simulink library "Tube_Alpha_sf"  (R2019b)
settings: Solver=ode45  StartTime=0.0  StopTime=10.0  RelTol=1e-3  EnableMultiTasking=on
undefined symbols (not defined in the file): Tube
libraries: simulink x1
settings Model: Creator=mbrauer  LastModifiedBy=bhisma
settings DataIOCC: LimitDataPoints=on  SaveFormat=Array  SignalLoggingSaveFormat=ModelDataLogs  ReturnWorkspaceOutputs=off
settings OptimizationCC: LifeSpan=inf
settings DebuggingCC: UnderspecifiedInitializationDetection=Classic  MergeDetectMultiDrivingBlocksExec=none  SolverPrmCheckMsg=warning  MultiTaskDSMMsg=warning  MultiTaskCondExecSysMsg=none  SFUnexpectedBacktrackingDiag=warning  SFNoUnconditionalDefaultTransitionDiag=warning  SFExecutionAtInitializationDiag=none  ArithmeticOperatorsInVariantConditions=warning
settings HardwareCC: ProdBitPerPointer=32  ProdBitPerSizeT=32  ProdBitPerPtrDiffT=32  ProdLargestAtomicFloat=None  ProdIntDivRoundTo=Undefined  ProdEndianess=Unspecified  ProdWordSize=32  ProdHWDeviceType=32-bit Generic
settings ModelReferenceCC: PropagateSignalLabelsOutOfModel=off
settings SFSimCC: SimUseLocalCustomCode=off  CustomCodeUndefinedFunction=UseInterfaceOnly
settings RTWCC: RTWUseLocalCustomCode=off
settings CodeAppCC: StateflowObjectComments=on
settings GRTTargetCC: TargetLangStandard=C89/C90 (ANSI)  GeneratePreprocessorConditionals=Disable all
settings ConfigComp: CovMetricSettings=dw  CovHtmlReporting=on  CovSaveCumulativeToWorkspaceVar=on  CovSaveSingleToWorkspaceVar=on  CovExternalEMLEnable=off

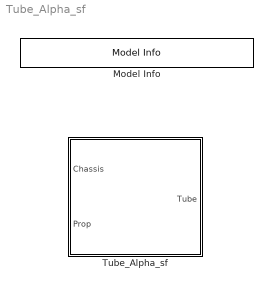
== system Tube_Alpha_sf ==
  Model Info : simulink/Model-Wide Utilities/Model Info  Frame=on  DisplayStringWithTags=Copyright 2013-2014 The MathWorks, Inc.  HorizontalTextAlignment=Center  LeftAlignmentValue=0.5
  Tube_Alpha_sf : Subsystem  VariantControl=VAR_Tube_Alpha

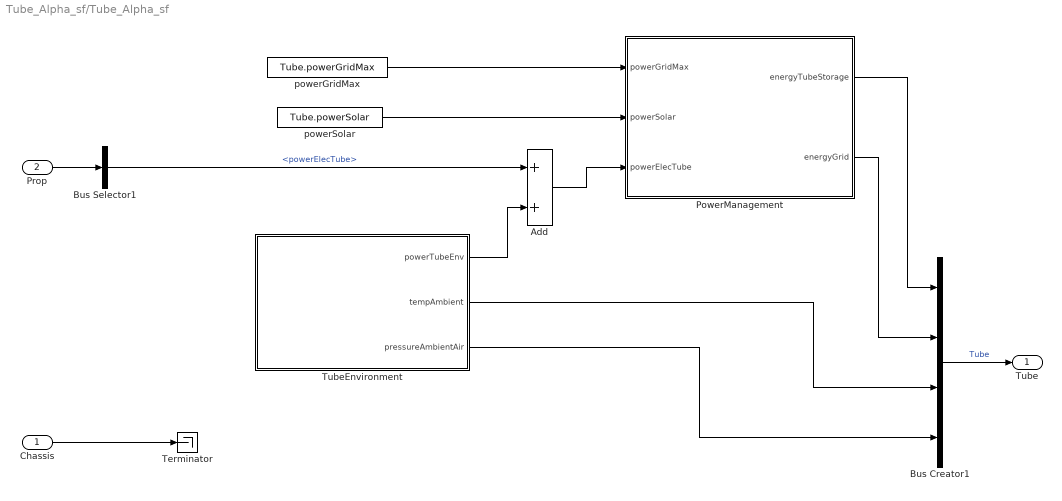
== system Tube_Alpha_sf/Tube_Alpha_sf ==
  Chassis : Inport
  Prop : Inport  Port=2
  Add : Sum
  Bus Creator1 : BusCreator  Inputs=4  NonVirtualBus=on
  Bus Selector1 : BusSelector  OutputSignals=powerElecTube
  PowerManagement : Subsystem
  Terminator : Terminator
  TubeEnvironment : Subsystem
  powerGridMax : Constant  Value=Tube.powerGridMax
  powerSolar : Constant  Value=Tube.powerSolar
  Tube : Outport
  wires:
  TubeEnvironment/2(tempAmbient) -> Bus Creator1/3
  Bus Creator1/1 -> Tube/1  "Tube"
  PowerManagement/1(energyTubeStorage) -> Bus Creator1/1
  Prop/1 -> Bus Selector1/1
  TubeEnvironment/1(powerTubeEnv) -> Add/2
  PowerManagement/2(energyGrid) -> Bus Creator1/2
  TubeEnvironment/3(pressureAmbientAir) -> Bus Creator1/4
  powerSolar/1 -> PowerManagement/2(powerSolar)
  powerGridMax/1 -> PowerManagement/1(powerGridMax)
  Bus Selector1/1 -> Add/1  "<powerElecTube>"
  Add/1 -> PowerManagement/3(powerElecTube)
  Chassis/1 -> Terminator/1

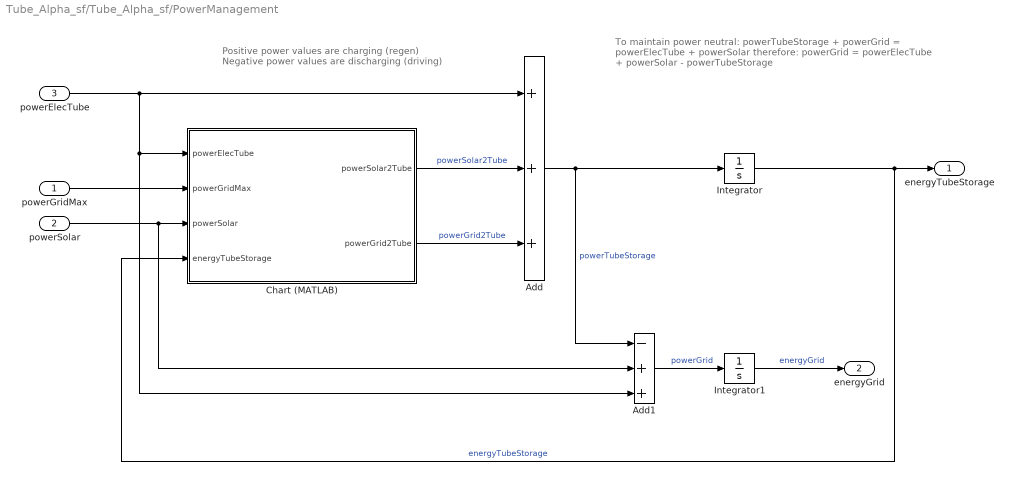
== system Tube_Alpha_sf/Tube_Alpha_sf/PowerManagement ==
  note: To maintain power neutral:
      | powerTubeStorage + powerGrid = powerElecTube + powerSolar
      |
      | therefore:
      | powerGrid = powerElecTube + powerSolar - powerTubeStorage
  note: Positive power values are charging (regen)
      | Negative power values are discharging (driving)
  powerGridMax : Inport
  powerSolar : Inport  Port=2
  powerElecTube : Inport  Port=3
  Add : Sum  Inputs=+++
  Add1 : Sum  Inputs=-++
  Chart (MATLAB) : Stateflow chart  TreatAsAtomicUnit=on
  Integrator : Integrator  InitialCondition=Tube.energyStorage
      settings: AttributesFormatString=IC = %<InitialCondition>
  Integrator1 : Integrator
      settings: AttributesFormatString=IC = %<InitialCondition>
  energyTubeStorage : Outport
  energyGrid : Outport  Port=2
  wires:
  Add/1 -> Integrator/1, Add1/1  "powerTubeStorage"
  Integrator1/1 -> energyGrid/1  "energyGrid"
  powerElecTube/1 -> Add1/3, Chart (MATLAB)/1(powerElecTube), Add/1
  Integrator/1 -> Chart (MATLAB)/4(energyTubeStorage), energyTubeStorage/1  "energyTubeStorage"
  powerGridMax/1 -> Chart (MATLAB)/2(powerGridMax)
  powerSolar/1 -> Chart (MATLAB)/3(powerSolar), Add1/2
  Chart (MATLAB)/1(powerSolar2Tube) -> Add/2  "powerSolar2Tube"
  Chart (MATLAB)/2(powerGrid2Tube) -> Add/3  "powerGrid2Tube"
  Add1/1 -> Integrator1/1  "powerGrid"

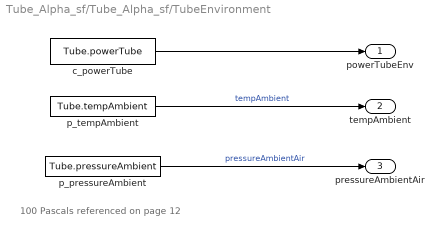
== system Tube_Alpha_sf/Tube_Alpha_sf/TubeEnvironment ==
  note: 100 Pascals referenced on page 12
  c_powerTube : Constant  Value=Tube.powerTube
  p_pressureAmbient : Constant  Value=Tube.pressureAmbient
  p_tempAmbient : Constant  Value=Tube.tempAmbient
  powerTubeEnv : Outport
  tempAmbient : Outport  Port=2
  pressureAmbientAir : Outport  Port=3
  wires:
  p_tempAmbient/1 -> tempAmbient/1  "tempAmbient"
  p_pressureAmbient/1 -> pressureAmbientAir/1  "pressureAmbientAir"
  c_powerTube/1 -> powerTubeEnv/1

== stateflow chart Tube_Alpha_sf/PowerManagement/Chart (MATLAB) ==
  state Default
    du: powerSolar2Tube = powerSolar;
    du: powerGrid2Tube =0;
  data: powerElecTube input; powerGridMax input; powerSolar input; powerSolar2Tube output; powerGrid2Tube output; energyTubeStorage input
